simulink model "controls"  (R2022a)
settings: Solver=ode3  StartTime=0.0  StopTime=10.0  FixedStep=0.001  RelTol=1e-3
undefined symbols (not defined in the file or in its folder): par
libraries: eeGeneralControl x11, simulink x9, matrix_library x3, dspinverses x1
settings Model: Creator=Matthias  LastModifiedBy=rjaneau
settings SolverCC: AlgebraicLoopSolver=TrustRegion
settings DataIOCC: ReturnWorkspaceOutputs=off
settings DebuggingCC: UnconnectedInputMsg=warning  UnconnectedOutputMsg=warning  UnconnectedLineMsg=warning  ModelReferenceExtraNoncontSigs=warning  SFMachineParentedDataDiag=warning  ArithmeticOperatorsInVariantConditions=warning
settings ModelReferenceCC: ModelReferenceNumInstancesAllowed=Single
settings SFSimCC: CustomCodeUndefinedFunction=UseInterfaceOnly

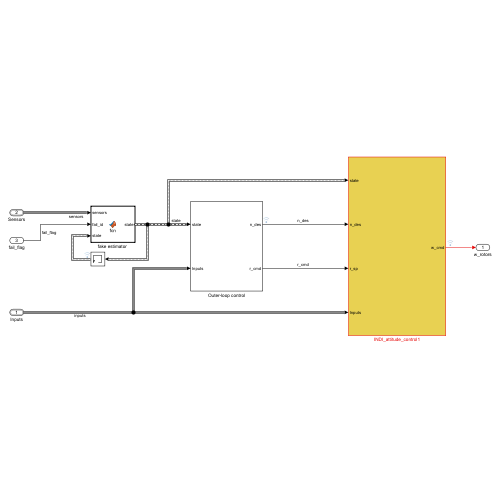
[thumbnail: Simulink's stored preview of the top-level diagram]
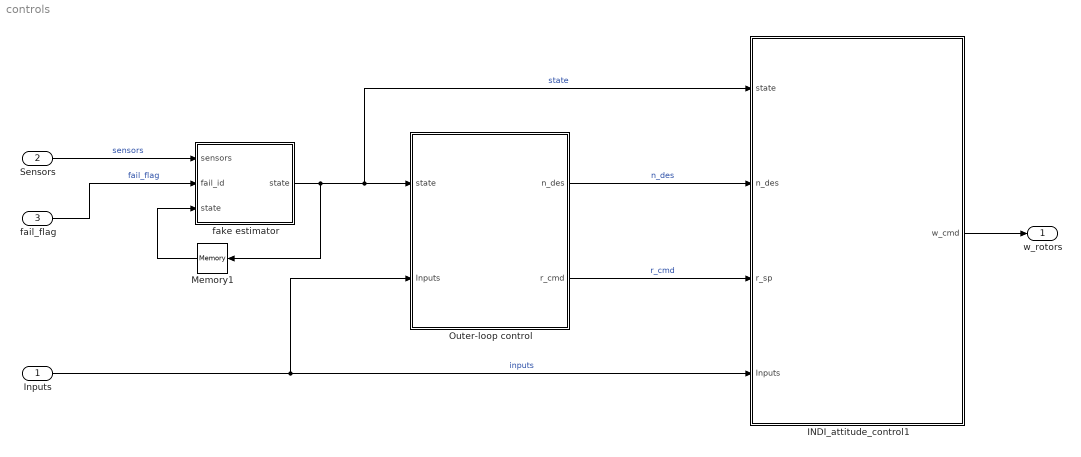
== system controls ==
  Inputs : Inport  OutDataTypeStr=Bus: inputsBus
  Sensors : Inport  Port=2  OutDataTypeStr=Bus: sensorsBus
  fail_flag : Inport  Port=3  OutDataTypeStr=double  PortDimensions=1
  INDI_attitude_control1 : Subsystem
  Memory1 : Memory
  Outer-loop control : Subsystem
  "fake estimator " : MATLAB Function  TreatAsAtomicUnit=on
  w_rotors : Outport  VectorParamsAs1DForOutWhenUnconnected=off
  wires:
  fail_flag/1 -> "fake estimator "/2(fail_id)  "fail_flag"
  Outer-loop control/2(r_cmd) -> INDI_attitude_control1/3(r_sp)  "r_cmd"
  "fake estimator "/1(state) -> Memory1/1, INDI_attitude_control1/1(state), Outer-loop control/1(state)  "state"
  Inputs/1 -> INDI_attitude_control1/4(Inputs), Outer-loop control/2(Inputs)  "inputs"
  INDI_attitude_control1/1(w_cmd) -> w_rotors/1
  Outer-loop control/1(n_des) -> INDI_attitude_control1/2(n_des)  "n_des"
  Memory1/1 -> "fake estimator "/3("state ")
  Sensors/1 -> "fake estimator "/1(sensors)  "sensors"

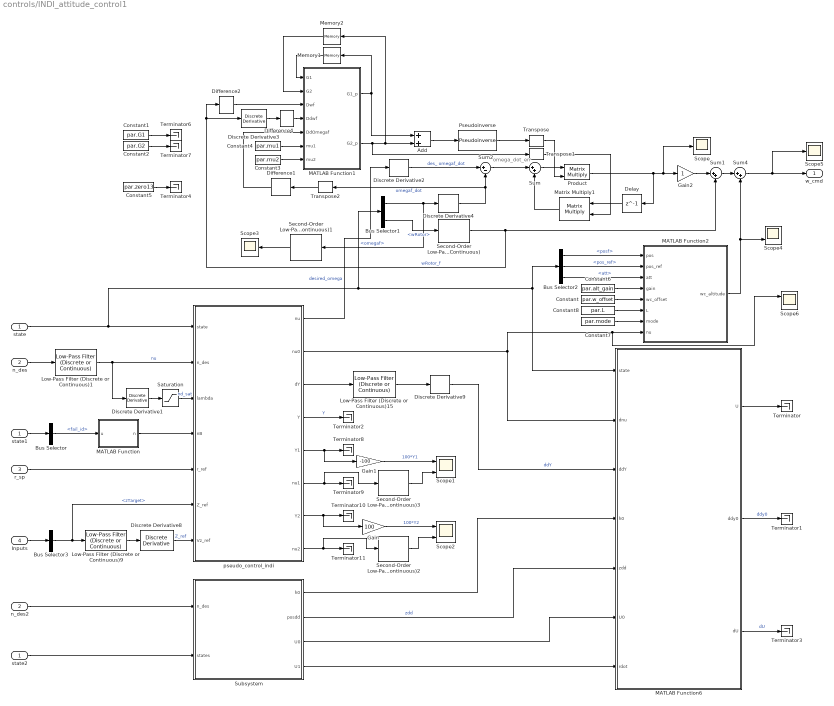
== system controls/INDI_attitude_control1 ==
  note: omega_dot_err
  state : Inport
  n_des : Inport  Port=2  PortDimensions=3
  r_sp : Inport  Port=3
  Inputs : Inport  Port=4
  Add : Sum
  Bus Selector : BusSelector  OutputSignals=fail_id
  Bus Selector1 : BusSelector  OutputSignals=omegaf,wRotor
  Bus Selector2 : BusSelector  OutputSignals=posf,pos_ref,att
  Bus Selector3 : BusSelector  OutputSignals=zTarget
  Constant : Constant  Value=par.w_offset
  Constant1 : Constant  Value=par.G1
  Constant2 : Constant  Value=par.G2
  Constant3 : Constant  Value=par.mu2
  Constant4 : Constant  Value=par.mu1
  Constant5 : Constant  Value=par.zero13
  Constant6 : Constant  Value=par.alt_gain
  Constant7 : Constant  Value=par.mode
  Constant8 : Constant  Value=par.L
  Delay : Delay  DelayLength=1  InitialCondition=0
  Difference1 : simulink/Discrete/Difference  ICPrevInput=0.0  OutMin=[]  OutMax=[]  OutDataType=fixdt(1, 16)  OutScaling=2^-10  DoSatur=off
  Difference2 : simulink/Discrete/Difference  ICPrevInput=0.0  OutMin=[]  OutMax=[]  OutDataType=fixdt(1, 16)  OutScaling=2^-10  DoSatur=off
  Difference4 : simulink/Discrete/Difference  ICPrevInput=0.0  OutMin=[]  OutMax=[]  OutDataType=fixdt(1, 16)  OutScaling=2^-10  DoSatur=off
  Discrete Derivative{1..4,8..9} (6 alike) : simulink/Discrete/Discrete Derivative  gainval=1.0  ICPrevScaledInput=0.0  OutMin=[]  OutMax=[]  OutDataType=fixdt(1, 16)  OutScaling=2^-10  DoSatur=off
  Gain : Gain  Gain=100
  Gain1 : Gain  Gain=-100
  Gain2 : Gain
  Low-Pass Filter (Discrete or Continuous)1 : eeGeneralControl/Low-Pass Filter (Discrete or Continuous)  K=1  T=par.t_indi  B=inf  A=-inf  init_option=Inherited from block input  x0=0  Ts=-1
  Low-Pass Filter (Discrete or Continuous)15 : eeGeneralControl/Low-Pass Filter (Discrete or Continuous)  K=1  T=par.t_indi  B=inf  A=-inf  init_option=Inherited from block input  x0=0  Ts=-1
  Low-Pass Filter (Discrete or Continuous)9 : eeGeneralControl/Low-Pass Filter (Discrete or Continuous)  K=1  T=par.t_indi  B=inf  A=-inf  init_option=Inherited from block input  x0=0  Ts=-1
  MATLAB Function : MATLAB Function  TreatAsAtomicUnit=on
  MATLAB Function1 : MATLAB Function  TreatAsAtomicUnit=on
  MATLAB Function2 : MATLAB Function  TreatAsAtomicUnit=on
  MATLAB Function6 : MATLAB Function  TreatAsAtomicUnit=on
  Matrix Multiply1 : Product  Multiplication=Matrix(*)
  Memory1 : Memory  InitialCondition=par.G1  LinearizeMemory=on
  Memory2 : Memory  InitialCondition=par.G2  LinearizeMemory=on
  Product : Product  Multiplication=Matrix(*)
  Pseudoinverse : dspinverses/Pseudoinverse  wanterr=off  SimulateUsing=Interpreted execution
      settings: SourceProductBaseCode=DS
  Saturation : Saturate
  Scope : Scope
  Scope{1..2,4,6} (4 alike) : Scope  NumInputPorts=2
  Scope3 : Scope
  Scope5 : Scope
  Second-Order Low-Pass Filter (Discrete or Continuous){,1..3} (4 alike) : eeGeneralControl/Second-Order Low-Pass Filter (Discrete or Continuous)  A1=0.022  A2=0.0004  init_option=Inherited from block input  x0=0  Ts=-1
      settings: SourceProductBaseCode=PS
  Subsystem : Subsystem
  Sum : Sum  Inputs=|++
  Sum1 : Sum  Inputs=|++
  Sum2 : Sum  Inputs=|+-
  Sum4 : Sum  Inputs=|++
  Terminator{,1..4,6..11} (11 alike) : Terminator
  Transpose : matrix_library/Transpose
      settings: SourceProductBaseCode=SL
  Transpose1 : matrix_library/Transpose
      settings: SourceProductBaseCode=SL
  Transpose2 : matrix_library/Transpose
      settings: SourceProductBaseCode=SL
  n_des2 : InportShadow  Port=2  PortDimensions=3
  pseudo_control_indi : MATLAB Function  TreatAsAtomicUnit=on
  state1 : InportShadow
  state2 : InportShadow
  w_cmd : Outport  VectorParamsAs1DForOutWhenUnconnected=off
  wires:
  MATLAB Function6/3(dU) -> Terminator3/1  "dU"
  Inputs/1 -> Bus Selector3/1
  r_sp/1 -> pseudo_control_indi/5(r_ref)
  Discrete Derivative8/1 -> pseudo_control_indi/7(Vz_ref)  "Z_ref"
  Bus Selector3/1 -> pseudo_control_indi/6(Z_ref), Low-Pass Filter (Discrete or Continuous)9/1  "<zTarget>"
  Low-Pass Filter (Discrete or Continuous)9/1 -> Discrete Derivative8/1
  MATLAB Function/1(n) -> pseudo_control_indi/4(nB)
  n_des/1 -> Low-Pass Filter (Discrete or Continuous)1/1
  pseudo_control_indi/3(dY) -> Low-Pass Filter (Discrete or Continuous)15/1
  Discrete Derivative9/1 -> MATLAB Function6/3(ddY)  "ddY"
  Low-Pass Filter (Discrete or Continuous)15/1 -> Discrete Derivative9/1
  n_des2/1 -> Subsystem/1(n_des)
  Subsystem/1(h0) -> MATLAB Function6/4(h0)
  Subsystem/2(posdd) -> MATLAB Function6/5(zdd)  "zdd"
  Subsystem/3(U0) -> MATLAB Function6/6(U0)
  Subsystem/4(U1) -> MATLAB Function6/7(rdot)
  Bus Selector/1 -> MATLAB Function/1(u)  "<fail_id>"
  state2/1 -> Subsystem/2(states)
  state/1 -> MATLAB Function6/1(state), Bus Selector2/1, Bus Selector1/1, pseudo_control_indi/1(state)
  state1/1 -> Bus Selector/1
  MATLAB Function6/2(ddy0) -> Terminator1/1  "ddy0"
  Discrete Derivative1/1 -> Saturation/1
  Saturation/1 -> pseudo_control_indi/3(lambda)  "nd_sat"
  MATLAB Function6/1(U) -> Terminator/1
  Matrix Multiply1/1 -> Sum/2
  Delay/1 -> Matrix Multiply1/1
  Product/1 -> Gain2/1, Scope/1, Delay/1
  Sum2/1 -> Sum/1
  pseudo_control_indi/2(nu0) -> Scope6/1, MATLAB Function2/8(nu), MATLAB Function6/2(dnu)
  Add/1 -> Pseudoinverse/1
  MATLAB Function1/2(G2_p) -> Transpose1/1, Memory2/1, Add/2
  Constant3/1 -> MATLAB Function1/7(mu2)
  Constant4/1 -> MATLAB Function1/6(mu1)
  Second-Order Low-Pass Filter (Discrete or Continuous)/1 -> Discrete Derivative3/1, Difference2/1, Sum1/2  "wRotor_f"
  Difference1/1 -> MATLAB Function1/5(DdOmegaf)
  Pseudoinverse/1 -> Transpose/1
  Sum/1 -> Product/1
  Transpose/1 -> Product/2
  Transpose1/1 -> Matrix Multiply1/2
  Transpose2/1 -> Difference1/1
  MATLAB Function1/1(G1_p) -> Memory1/1, Add/1
  Discrete Derivative4/1 -> Sum2/2, Transpose2/1  "omegaf_dot"
  Bus Selector1/2 -> Second-Order Low-Pass Filter (Discrete or Continuous)/1  "<wRotor>"
  Low-Pass Filter (Discrete or Continuous)1/1 -> Discrete Derivative1/1, pseudo_control_indi/2(n_des)  "nu"
  Difference2/1 -> MATLAB Function1/3(Dwf)
  Constant1/1 -> Terminator6/1
  Constant2/1 -> Terminator7/1
  Memory2/1 -> MATLAB Function1/2(G2)
  Memory1/1 -> MATLAB Function1/1(G1)
  Constant5/1 -> Terminator4/1
  Sum4/1 -> Scope5/1, w_cmd/1
  Sum1/1 -> Sum4/1
  Constant6/1 -> MATLAB Function2/4(gain)
  MATLAB Function2/1(wc_altitude) -> Scope4/2, Sum4/2
  Constant/1 -> MATLAB Function2/5(wc_offset)
  pseudo_control_indi/5(Y1) -> Terminator8/1, Gain1/1
  pseudo_control_indi/4(Y) -> Terminator2/1  "Y"
  pseudo_control_indi/8(nu2) -> Terminator11/1, Second-Order Low-Pass Filter (Discrete or Continuous)2/1
  pseudo_control_indi/6(nu1) -> Second-Order Low-Pass Filter (Discrete or Continuous)3/1, Terminator9/1
  pseudo_control_indi/7(Y2) -> Terminator10/1, Gain/1
  Second-Order Low-Pass Filter (Discrete or Continuous)1/1 -> Scope3/1
  Bus Selector1/1 -> Second-Order Low-Pass Filter (Discrete or Continuous)1/1, Discrete Derivative4/1  "<omegaf>"
  Bus Selector2/2 -> MATLAB Function2/2(pos_ref)  "<pos_ref>"
  Discrete Derivative2/1 -> Sum2/1  "des_ omegaf_dot"
  Constant7/1 -> MATLAB Function2/7(mode)
  Bus Selector2/3 -> MATLAB Function2/3(att)  "<att>"
  Constant8/1 -> MATLAB Function2/6(L)
  Gain/1 -> Scope2/1  "100*Y2"
  Gain1/1 -> Scope1/1  "100*Y1"
  pseudo_control_indi/1(nu) -> Discrete Derivative2/1  "desired_omega"
  Discrete Derivative3/1 -> Difference4/1
  Difference4/1 -> MATLAB Function1/4(Ddwf)
  Bus Selector2/1 -> MATLAB Function2/1(pos)  "<posf>"
  Second-Order Low-Pass Filter (Discrete or Continuous)2/1 -> Scope2/2
  Second-Order Low-Pass Filter (Discrete or Continuous)3/1 -> Scope1/2
  Gain2/1 -> Sum1/1

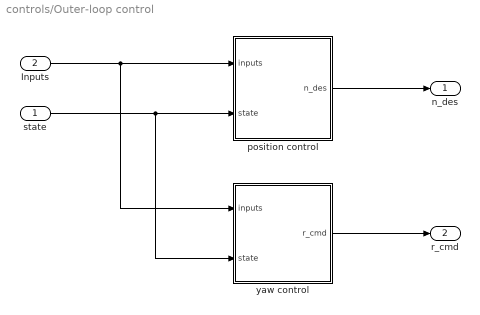
== system controls/Outer-loop control ==
  state : Inport
  Inputs : Inport  Port=2
  position control : MATLAB Function  TreatAsAtomicUnit=on
  yaw control : MATLAB Function  TreatAsAtomicUnit=on
  n_des : Outport  VectorParamsAs1DForOutWhenUnconnected=off
  r_cmd : Outport  Port=2  VectorParamsAs1DForOutWhenUnconnected=off
  wires:
  yaw control/1(r_cmd) -> r_cmd/1
  Inputs/1 -> yaw control/1(inputs), position control/1(inputs)
  state/1 -> yaw control/2(state), position control/2(state)
  position control/1(n_des) -> n_des/1

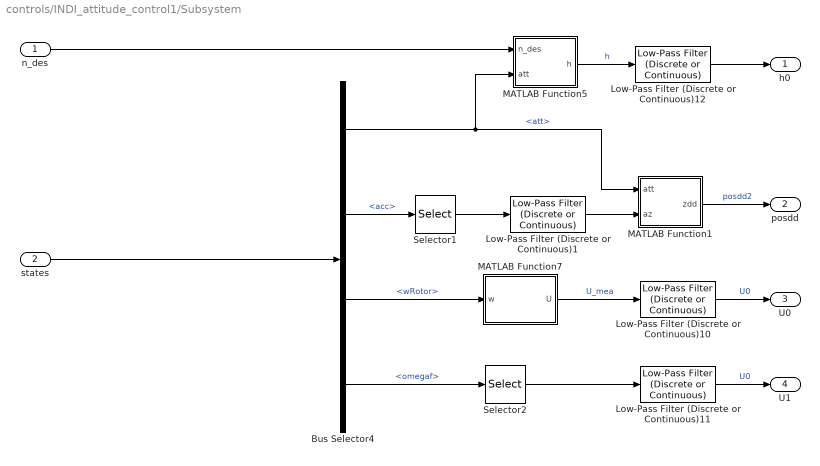
== system controls/INDI_attitude_control1/Subsystem ==
  n_des : Inport
  states : Inport  Port=2
  Bus Selector4 : BusSelector  OutputSignals=att,acc,wRotor,omegaf
  Low-Pass Filter (Discrete or Continuous){1,10..12} (4 alike) : eeGeneralControl/Low-Pass Filter (Discrete or Continuous)  K=1  T=par.t_indi  B=inf  A=-inf  init_option=Inherited from block input  x0=0  Ts=-1
  MATLAB Function1 : MATLAB Function  TreatAsAtomicUnit=on
  MATLAB Function5 : MATLAB Function  TreatAsAtomicUnit=on
  MATLAB Function7 : MATLAB Function  TreatAsAtomicUnit=on
  Selector1 : Selector  InputPortWidth=3  IndexOptions=Index vector (dialog)  Indices=3  OutputSizes=1
  Selector2 : Selector  InputPortWidth=3  IndexOptions=Index vector (dialog)  Indices=3  OutputSizes=1
  h0 : Outport  VectorParamsAs1DForOutWhenUnconnected=off
  posdd : Outport  Port=2  VectorParamsAs1DForOutWhenUnconnected=off
  U0 : Outport  Port=3  VectorParamsAs1DForOutWhenUnconnected=off
  U1 : Outport  Port=4  VectorParamsAs1DForOutWhenUnconnected=off
  wires:
  Bus Selector4/4 -> Selector2/1  "<omegaf>"
  Bus Selector4/3 -> MATLAB Function7/1(w)  "<wRotor>"
  Bus Selector4/1 -> MATLAB Function5/2(att), MATLAB Function1/1(att)  "<att>"
  states/1 -> Bus Selector4/1
  MATLAB Function5/1(h) -> Low-Pass Filter (Discrete or Continuous)12/1  "h"
  Selector2/1 -> Low-Pass Filter (Discrete or Continuous)11/1
  MATLAB Function7/1(U) -> Low-Pass Filter (Discrete or Continuous)10/1  "U_mea"
  Low-Pass Filter (Discrete or Continuous)10/1 -> U0/1  "U0"
  Low-Pass Filter (Discrete or Continuous)11/1 -> U1/1  "U0"
  Low-Pass Filter (Discrete or Continuous)12/1 -> h0/1
  n_des/1 -> MATLAB Function5/1(n_des)
  Bus Selector4/2 -> Selector1/1  "<acc>"
  Selector1/1 -> Low-Pass Filter (Discrete or Continuous)1/1
  Low-Pass Filter (Discrete or Continuous)1/1 -> MATLAB Function1/2(az)
  MATLAB Function1/1(zdd) -> posdd/1  "posdd2"

== matlab function controls/INDI_attitude_control1/Subsystem/MATLAB Function1 ==
  data: att input; az input; zdd output
function zdd = fcn(att,az)

phi = att(1);
theta = att(2);

zdd = az*cos(theta)*cos(phi) + 9.8124;

== matlab function controls/INDI_attitude_control1/Subsystem/MATLAB Function5 ==
  data: n_des input; att input; h output
function h = fcn(n_des, att)

phi = att(1);
theta = att(2);
psi = att(3);

R_IB = [cos(psi)*cos(theta) , cos(psi)*sin(theta)*sin(phi)-sin(psi)*cos(phi), cos(psi)*sin(theta)*cos(phi)+sin(psi)*sin(phi);
        sin(psi)*cos(theta) , sin(psi)*sin(theta)*sin(phi)+cos(psi)*cos(phi), sin(psi)*sin(theta)*cos(phi)-cos(psi)*sin(phi);
        -sin(theta)          , cos(theta)*sin(phi)                          , cos(theta)*cos(phi)                          ];

h = R_IB \ n_des;

== matlab function controls/INDI_attitude_control1/Subsystem/MATLAB Function7 ==
  data: w input; U output
function U = omega2U(w)
%#codegen

U = zeros(4,1);
U(1) = w(1)^2;
U(2) = w(2)^2;
U(3) = w(3)^2;
U(4) = w(4)^2;
end

== matlab function controls/INDI_attitude_control1/pseudo_control_indi ==
  data: nu output; nu0 output; state input; n_des input; lambda input; nB input; r_ref input; Z_ref input; Vz_ref input; par parameter; dY output; Y output; Y1 output; nu1 output; Y2 output; nu2 output
function [nu,nu0,dY, Y,Y1,nu1,Y2,nu2] = pseudo_control_att_indi(state, n_des, lambda, nB, r_ref, Z_ref, Vz_ref, par)

[nu,nu0, dY, Y] = pseudo_control_att_indi(state, n_des, lambda, nB, r_ref, Z_ref, Vz_ref, par);

Y1=Y(1);
Y2=Y(2);
nu1=nu(1);
nu2=nu(2);

end

== matlab function controls/INDI_attitude_control1/MATLAB Function1 ==
  data: G1_p output; G2_p output; G1 input; G2 input; Dwf input; Ddwf input; DdOmegaf input; mu1 input; mu2 input
function [G1_p,G2_p]= G_update(G1,G2,Dwf,Ddwf,DdOmegaf,mu1,mu2)

%% Dimensions %%
% G_km = [[3x4] [3x4]]
% mu1 = [4x4]
% mu2 = [3x3]
% Dwf, Ddwf = [1x4]
% DdOmegaf = [3x1]

%% G Update %%

%G_km = [G1 G2]; 
%G_k = G_km - mu2*(G_km*[transpose(Dwf);transpose(Ddwf)] - DdOmegaf)*[Dwf Ddwf]*mu1;
%G1_p=G_k(1);
%G2_p=G_k(2);

mu11 = mu1;
mu12 = 0.5*mu1;

G1_p = G1 - mu2*(G1*transpose(Dwf)+G2*transpose(Ddwf) - DdOmegaf)*Dwf*mu11; 
G2_p = G2 - mu2*(G1*transpose(Dwf)+G2*transpose(Ddwf) - DdOmegaf)*Ddwf*mu12; 
%[3x4] = [3x4] - [3x3]*([3x4]*[4x1]+[3x4]*[4x1] - [3x1])*[1x4]*[4x4]

%disp(G2_p);

== matlab function controls/Outer-loop control/position control ==
  data: inputs input Bus: inputsBus; n_des output size=[1 3]; state input Bus: stateBus; par parameter
function n_des   = positionControl(inputs, state, par)

[n_des] = URpositionControl(inputs, state, par);

end

== matlab function controls/Outer-loop control/yaw control ==
  data: inputs input Bus: inputsBus; r_cmd output; state input Bus: stateBus; par parameter
function r_cmd = yawControl(inputs, state, par)

[r_cmd] = URYawControl(inputs, state, par);

end

== matlab function controls/fake estimator  ==
  data: sensors input; fail_id input; state input Bus: stateBus; state output
function state = fcn(sensors, fail_id, state)

state = UREstimators(sensors, state, fail_id);

end

== matlab function controls/INDI_attitude_control1/MATLAB Function2 ==
  data: wc_altitude output; pos input; pos_ref input; att input; gain input; wc_offset input; L input; mode input; nu input
function wc_altitude  = altitude_cmd(pos,pos_ref,att,gain,wc_offset,L,mode,nu)

if mode==1
    cmd = gain*(pos(3)-pos_ref(3))+wc_offset;
else
    ddz_ctrl_input=nu(1);
    cmd = -gain*ddz_ctrl_input;
end

wc_altitude = [cmd,cmd,cmd,cmd];

% Adjustments based on roll and pitch angle (comment to disable)

phi = att(1);
theta = att(2);

%V1
% corrective_roll = 1000* L * nu(1) * sin(theta);
% corrective_pitch = 1000* L * nu(1) * sin(phi);
% wc_altitude = wc_altitude + [corrective_roll,-corrective_pitch,corrective_roll,-corrective_pitch];

%V2
% wc_altitude = abs(cos(theta)*cos(phi))*wc_altitude;

if (abs(theta)>pi/2) || (abs(phi)>pi/2) 
    wc_altitude=[0,0,0,0];
    %disp('upside down !')
end

if wc_altitude>[1200,1200,1200,1200]
    wc_altitude=[1200,1200,1200,1200];
end

== matlab function controls/INDI_attitude_control1/MATLAB Function ==
  data: u input; n output; par parameter
function n = fcn(u,par)

a = par.axis_tilt;

if par.DRF_enable == 0 || par.DRF_enable == 1 
    if u == 1
       n = [-a, a, -1];   
    elseif u == 2
       n = [-a, -a, -1];
    elseif u == 3
       n = [a, -a, -1];
    elseif u == 4
       n = [a, a, -1];
    else
       n = [0, 0, -1];    
    end
else
   n = [0, 0, -1];
end

== matlab function controls/INDI_attitude_control1/MATLAB Function6 ==
  data: state input; dnu input; ddY input; h0 input; zdd input; U0 input; rdot input; U output; par parameter; ddy0 output; dU output
function [U,ddy0,dU]  =  allocation_att_indi(state, dnu, ddY, h0, zdd, U0, rdot, par)
    [U,ddy0,dU]  =  allocation_att_indi(state, dnu, ddY, h0, zdd, U0, rdot, par);
end
